simulink model "twodofsim"  (R2021a)
settings: Solver=VariableStepAuto  StartTime=0.0  StopTime=10.0  RelTol=1e-3
settings Model: Creator=cjobr  LastModifiedBy=cjobr

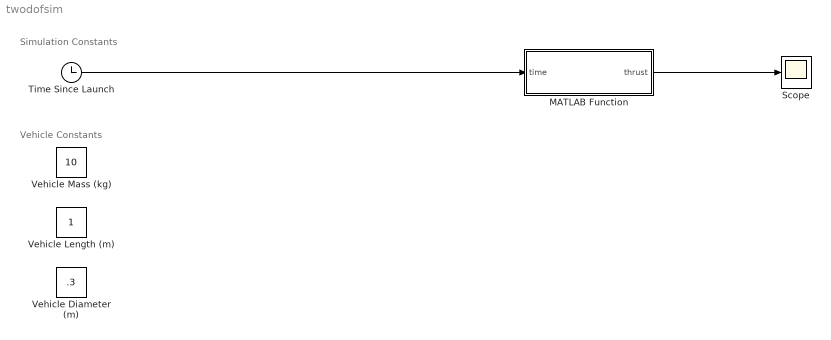
== system twodofsim ==
  note: Simulation Constants
  note: Vehicle Constants
  MATLAB Function : MATLAB Function  TreatAsAtomicUnit=on
  Scope : Scope
  Time Since Launch : Clock
  Vehicle Diameter (m) : Constant  Value=.3
  Vehicle Length (m) : Constant
  Vehicle Mass (kg) : Constant  Value=10
  wires:
  Time Since Launch/1 -> MATLAB Function/1(time)
  MATLAB Function/1(thrust) -> Scope/1

== matlab function twodofsim/MATLAB Function ==
  data: time input; thrust output
function thrust = getThrustData(time)
%Increase discrete data resolution by factor of Res
Res = 20;

%Create more detailed matrices of data
time_extended = interp(ThrustData(:,1),Res);
thrust_extended = interp(ThrustData(:,2),Res);
burntime = time_extended(end);

if(time < burntime)
    %Search for discrete increment of time that is closest to inputted time
    [minValue,closestIndex] = min(abs(time_extended-time));
    %return corresponding value of thrust
    thrust = thrust_extended(closestIndex);
else
    %if motor has burned out assume thrust is 0
    thrust = 0;
end

end
